simulink model "sf_example"  (R2018a)
settings: Solver=VariableStepAuto  StartTime=0.0  StopTime=10.0  RelTol=1e-3
settings Model: Creator=root  LastModifiedBy=BEAR
settings CodeAppCC: StateflowObjectComments=on

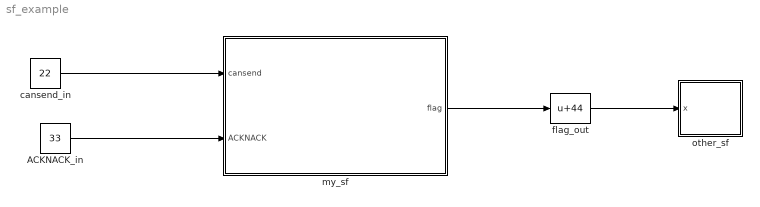
== system sf_example ==
  ACKNACK_in : Constant  Value=33
  cansend_in : Constant  Value=22
  flag_out : Bias  Bias=44
  my_sf : Stateflow chart  TreatAsAtomicUnit=on
  other_sf : Stateflow chart  TreatAsAtomicUnit=on
  wires:
  cansend_in/1 -> my_sf/1(cansend)
  ACKNACK_in/1 -> my_sf/2(ACKNACK)
  my_sf/1(flag) -> flag_out/1
  flag_out/1 -> other_sf/1(x)

== stateflow chart sf_example/other_sf ==
  state On
    en: x = 1
    du: x = 2
    ex: x = 3
    state Mid
      en: x = 4
      du: x = 5
      ex: x = 6
      state In
        en: x = 7
        du: x = 8
        ex: x = 9
      (default) -> On.Mid.In
    (default) -> Mid
  state Off
    en: x = 12
    du: x = 13
    ex: x = 14
    state In
      en: x = 16
      du: x = 17
      ex: x = 18
      state AND0 [parallel]
        settings: executionOrder=2
      state AND1 [parallel]
        settings: executionOrder=1
    (default) -> Off.In
  (default) -> On : {x = 0}
  On -> (junction 15) : [x>=3]{x=19}
  (junction 15) -> Off [order 1] : [x<10]{x=21}/{x=22}
  (junction 15) -> Off.In [order 2] : [x>=10]{x=23}/{x=24}
  Mid -> Off.In : [x == 2]{x = 10}/{x = 11}
  data: x input

== stateflow chart sf_example/my_sf ==
  state repairing
    during:flag=0
  state must_repair
    during:flag=1;
  state waiting
    during:flag=1;
  repairing -> repairing [order 1] : [cansend]/{re_changes = re_changes - 1}
  must_repair -> repairing [order 1] : after(ResponseDelay,sec)
  must_repair -> must_repair [order 2] : [ACKNACK]/{re_changes = re_changes + 1}
  repairing -> waiting [order 2] : [re_changes==0]
  waiting -> must_repair [order 2] : [re_changes>0]
  (default) -> waiting : {re_changes=0}
  waiting -> waiting [order 1] : [ACKNACK]/{re_changes = re_changes + 1}
  data: flag output; cansend input; re_changes local; ACKNACK input; ResponseDelay constant double
